simulink subsystem "final_value_generator"  (R2019b)
settings: Solver=VariableStepAuto  StartTime=0.0  StopTime=10.0  RelTol=1e-3
model mask{checkpoints=0, counter_max=0}
  mask prompts: counter_max "Number of transepts"
undefined symbols (not defined in the file): distance, pylonCenter
settings Model: Creator=andrea  LastModifiedBy=andrea

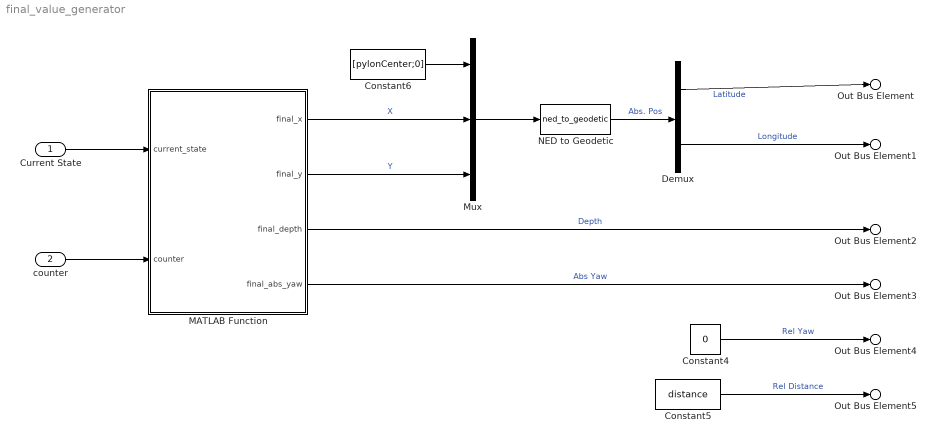
== system final_value_generator ==
  Current State : Inport
  counter : Inport  Port=2
  Constant4 : Constant  Value=0
  Constant5 : Constant  Value=distance
  Constant6 : Constant  Value=[pylonCenter;0]
  Demux : Demux  Outputs=2
  MATLAB Function : MATLAB Function  TreatAsAtomicUnit=on
  Mux : Mux  Inputs=3
  NED to Geodetic : MATLABFcn  MATLABFcn=ned_to_geodetic
  Out Bus Element : Outport  PortName=Final Value Bus  Element=Latitude
  Out Bus Element1 : Outport  PortName=Final Value Bus  Element=Longitude
  Out Bus Element2 : Outport  PortName=Final Value Bus  Element=Depth
  Out Bus Element3 : Outport  PortName=Final Value Bus  Element=Abs Yaw
  Out Bus Element4 : Outport  PortName=Final Value Bus  Element=Rel Yaw
  Out Bus Element5 : Outport  PortName=Final Value Bus  Element=Rel Distance
  wires:
  counter/1 -> MATLAB Function/2(counter)
  Current State/1 -> MATLAB Function/1(current_state)
  MATLAB Function/1(final_x) -> Mux/2  "X"
  MATLAB Function/2(final_y) -> Mux/3  "Y"
  Mux/1 -> NED to Geodetic/1
  Constant6/1 -> Mux/1
  NED to Geodetic/1 -> Demux/1  "Abs. Pos"
  Constant5/1 -> Out Bus Element5/1  "Rel Distance"
  Constant4/1 -> Out Bus Element4/1  "Rel Yaw"
  MATLAB Function/4(final_abs_yaw) -> Out Bus Element3/1  "Abs Yaw"
  MATLAB Function/3(final_depth) -> Out Bus Element2/1  "Depth"
  Demux/2 -> Out Bus Element1/1  "Longitude"
  Demux/1 -> Out Bus Element/1  "Latitude"

== matlab function final_value_generator/MATLAB Function ==
  data: current_state input; final_x output; counter input; final_y output; final_depth output; final_abs_yaw output; counter_max parameter; checkpoints parameter
function [final_x, final_y, final_depth, final_abs_yaw] = fcn(current_state, counter, counter_max, checkpoints)

row_index = checkpoint_row_index(current_state, counter, counter_max);
if row_index == -1
    final_x = 0;
    final_y = 0;
    final_depth = 0;
    final_abs_yaw = 0;
else
    final_x = checkpoints(row_index, 5);
    final_y = checkpoints(row_index, 6);
    final_depth = checkpoints(row_index, 7);
    final_abs_yaw = checkpoints(row_index, 8);
end
